simulink model "Steering"  (R2016a)
settings: Solver=FixedStepAuto  StartTime=0.0  StopTime=10  FixedStep=0.1  RelTol=1e-3
libraries: simulink x1
settings Model: Creator=krentzts  LastModifiedBy=krentzts
settings SolverCC: AlgebraicLoopSolver=LineSearch

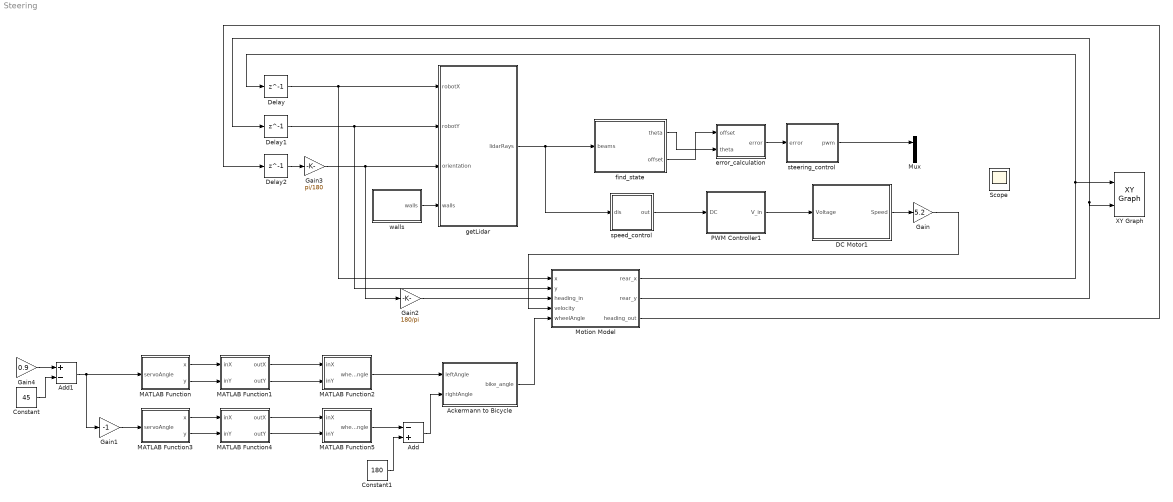
== system Steering ==
  Ackermann to Bicycle : MATLAB Function  TreatAsAtomicUnit=on
  Add : Sum  Inputs=-+
  Add1 : Sum  Inputs=+-
  Constant : Constant  Value=45
  Constant1 : Constant  Value=180
  DC Motor1 : Subsystem  mask{K=0.01, J=0.01, b=0.1, R=1, L=0.5}
      mask prompts: K "Ke (V/rad/sec), Kt (N.m/Amp)"; J "J (kg.m^2)"; b "b (N.m.s)"; R "R (Ohm)"; L "L (H)"
  Delay : Delay  DelayLength=1  InitialCondition=2
  Delay1 : Delay  DelayLength=1  InitialCondition=33
  Delay2 : Delay  DelayLength=1  InitialCondition=-20
  Gain : Gain  Gain=5.2
  Gain1 : Gain  Gain=-1
  Gain2 : Gain  Gain=180/pi
  Gain3 : Gain  Gain=pi/180
  Gain4 : Gain  Gain=0.9
  MATLAB Function : MATLAB Function  TreatAsAtomicUnit=on
  MATLAB Function1 : MATLAB Function  TreatAsAtomicUnit=on
  MATLAB Function2 : MATLAB Function  TreatAsAtomicUnit=on
  MATLAB Function3 : MATLAB Function  TreatAsAtomicUnit=on
  MATLAB Function4 : MATLAB Function  TreatAsAtomicUnit=on
  MATLAB Function5 : MATLAB Function  TreatAsAtomicUnit=on
  Motion Model : MATLAB Function  TreatAsAtomicUnit=on
  Mux : Mux  Inputs=2
  PWM Controller1 : Subsystem  mask{V=5}
      mask prompts: V "Maximum Voltage (V)"
  Scope : Scope
  XY Graph : simulink/Sinks/XY Graph  xmin=-1  xmax=1001  ymin=0  ymax=61  st=-1
  error_calculation : MATLAB Function  TreatAsAtomicUnit=on
  find_state : MATLAB Function  TreatAsAtomicUnit=on
  getLidar : MATLAB Function  TreatAsAtomicUnit=on
  speed_control : Stateflow chart  TreatAsAtomicUnit=on
  steering_control : Subsystem
  walls : MATLAB Function  TreatAsAtomicUnit=on
  wires:
  MATLAB Function/1(x) -> MATLAB Function1/1(inX)
  MATLAB Function/2(y) -> MATLAB Function1/2(inY)
  MATLAB Function1/1(outX) -> MATLAB Function2/1(inX)
  MATLAB Function1/2(outY) -> MATLAB Function2/2(inY)
  MATLAB Function2/1(wheelAngle) -> Ackermann to Bicycle/1(leftAngle)
  walls/1(walls) -> getLidar/4(walls)
  getLidar/1(lidarRays) -> find_state/1(beams), speed_control/1(dis)
  find_state/1(theta) -> error_calculation/2(theta)
  find_state/2(offset) -> error_calculation/1(offset)
  error_calculation/1(error) -> steering_control/1(error)
  PWM Controller1/1(V_in) -> DC Motor1/1(Voltage)
  DC Motor1/1(Speed) -> Gain/1
  Gain/1 -> Motion Model/4(velocity)
  Ackermann to Bicycle/1(bike_angle) -> Motion Model/5(wheelAngle)
  MATLAB Function3/1(x) -> MATLAB Function4/1(inX)
  MATLAB Function3/2(y) -> MATLAB Function4/2(inY)
  MATLAB Function4/1(outX) -> MATLAB Function5/1(inX)
  MATLAB Function4/2(outY) -> MATLAB Function5/2(inY)
  Gain1/1 -> MATLAB Function3/1(servoAngle)
  Add/1 -> Ackermann to Bicycle/2(rightAngle)
  MATLAB Function5/1(wheelAngle) -> Add/1
  Constant1/1 -> Add/2
  Gain2/1 -> Motion Model/3(heading_in)
  Motion Model/1(rear_x) -> Delay/1, XY Graph/1
  Motion Model/2(rear_y) -> XY Graph/2, Delay1/1
  Gain4/1 -> Add1/1
  Constant/1 -> Add1/2
  Add1/1 -> MATLAB Function/1(servoAngle), Gain1/1
  speed_control/1(out) -> PWM Controller1/1(DC)
  Delay2/1 -> Gain3/1
  Gain3/1 -> getLidar/3(orientation), Gain2/1
  Delay1/1 -> getLidar/2(robotY), Motion Model/2(y)
  Delay/1 -> getLidar/1(robotX), Motion Model/1(x)
  Motion Model/3(heading_out) -> Delay2/1
  steering_control/1(pwm) -> Mux/1

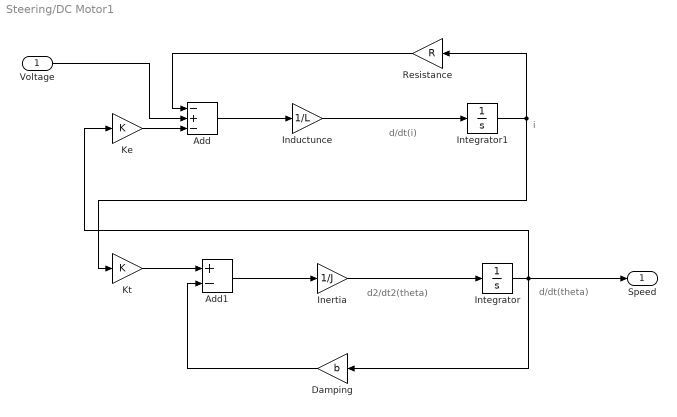
== system Steering/DC Motor1 ==
  note: d/dt(theta)
  note: i
  note: d2/dt2(theta)
  note: d/dt(i)
  Voltage : Inport
  Add : Sum  Inputs=-+-
  Add1 : Sum  Inputs=+-
  Damping : Gain  Gain=b
  Inductunce : Gain  Gain=1/L
  Inertia : Gain  Gain=1/J
  Integrator : Integrator
  Integrator1 : Integrator
  Ke : Gain  Gain=K
  Kt : Gain  Gain=K
  Resistance : Gain  Gain=R
  Speed : Outport
  wires:
  Kt/1 -> Add1/1
  Ke/1 -> Add/3
  Resistance/1 -> Add/1
  Voltage/1 -> Add/2
  Inductunce/1 -> Integrator1/1
  Integrator1/1 -> Resistance/1, Kt/1
  Inertia/1 -> Integrator/1
  Integrator/1 -> Speed/1, Damping/1, Ke/1
  Add/1 -> Inductunce/1
  Add1/1 -> Inertia/1
  Damping/1 -> Add1/2

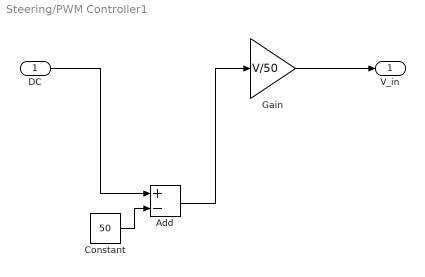
== system Steering/PWM Controller1 ==
  DC : Inport
  Add : Sum  Inputs=+-
  Constant : Constant  Value=50
  Gain : Gain  Gain=V/50
  V_in : Outport
  wires:
  Gain/1 -> V_in/1
  Constant/1 -> Add/2
  Add/1 -> Gain/1
  DC/1 -> Add/1

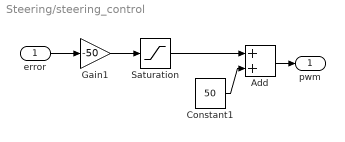
== system Steering/steering_control ==
  error : Inport
  Add : Sum
  Constant1 : Constant  Value=50
  Gain1 : Gain  Gain=-50
  Saturation : Saturate  UpperLimit=50  LowerLimit=-50
  pwm : Outport
  wires:
  error/1 -> Gain1/1
  Add/1 -> pwm/1
  Saturation/1 -> Add/1
  Gain1/1 -> Saturation/1
  Constant1/1 -> Add/2

== matlab function Steering/MATLAB Function1 ==
  data: inX input; outX output; inY input; outY output
function [outX,outY]  = pivotArm(inX,inY)
%#codegen
D = hypot(-1 - inX, -5 - inY);
theta1 = acosd((3.64^2 - 2^2 - D^2)/(-2*2*D));
theta2 = acosd((1+inX)/D);
thetaTotal = 360 - theta1 - theta2;

outLegAngle = thetaTotal - 180 + tand(1/2);

outX = -1 + sqrt(5)*cosd(outLegAngle);
outY = -5 + sqrt(5)*sind(outLegAngle);

== matlab function Steering/MATLAB Function ==
  data: x output; servoAngle input; y output
function [x,y] = servoHorn(servoAngle)
%#codegen

y = -7.07 + sind(270 - servoAngle);
x = 2.4813 + cosd(270 - servoAngle);

== matlab function Steering/MATLAB Function2 ==
  data: inX input; wheelAngle output; inY input
function wheelAngle = knuckle(inX,inY)
%#codegen
D = hypot(-10.5 - inX,0 - inY);
theta1 = acosd((9.2^2 - 1.5811^2 - D^2)/(-2*1.5811*D));
theta2 = acosd((10.5+inX)/D);
thetaTotal = 360 - theta1 - theta2;
wheelAngle = thetaTotal - 283.9 + 90;

== matlab function Steering/walls ==
  data: walls output
function walls = fcn()
walls=[1 1 1000 1;1 60 1000 60];
end

== matlab function Steering/getLidar ==
  data: robotX input; lidarRays output; robotY input; orientation input; walls input
function lidarRays = fcn(robotX,robotY,orientation,walls)

numLines = 512;
lidarRange = 60;

%Create rays matrix
lidarRays=zeros(numLines,2);
t = linspace(0,2*pi,numLines+1);
for i = 1:(length(t)-1);
    lidarRays(i,1) = lidarRange;
    lidarRays(i,2) = t(i);
end

[numWalls,~] = size(walls);
[numRays,~] = size(lidarRays);

%For each LIDAR ray...
for i = 1:numRays
    
    %Find its ending coordinate
    X = robotX + lidarRange*cos(t(i)+orientation);
    Y = robotY + lidarRange*sin(t(i)+orientation);
    
    %Find standard form of LIDAR ray
    R = [robotX robotY ; X Y];
    Q = inv(R)*[1;1];
    
    %For each wall...
    for j = 1:numWalls
        
        %Find standard form of wall
        P = [walls(j,1:2) ; walls(j,3:4)];
        O = inv(P)*[1;1];
        
        %Find intersection of wall and LIDAR ray
        INT = inv([Q';O'])*[1;1];
        intX = INT(1);  % x coordinate of intersection
        intY = INT(2);  % y coordinate of intersection
        
        %Check that intersection actually occurs within the
        %bounds of the LIDAR ray and wall
        if ((isBetween(intY,robotY,Y) == 1) && ...
            (isBetween(intX,robotX,X) == 1) && ...
            (isBetween(intX,walls(j,1),walls(j,3)) == 1) && ...
            (isBetween(intY,walls(j,2),walls(j,4)) == 1))
%             disp('INTERSECTION')
            temp = hypot((intX-robotX),(intY-robotY));
            
            %Clip ranges beyond max sensitivity
            if(temp > lidarRange)
                temp = lidarRange;
            end
            
            %Only store the minimum range for each wall
            if (lidarRays(i,1) > temp)
                lidarRays(i,1) = temp;
            end
        else
%             disp('NOPE')
        end
    end
end

== matlab function Steering/find_state ==
  data: theta output; beams input; offset output
function [theta,offset]  = fcn(beams)
step=2*pi/length(beams);
theta=0;
[~,minimum]=min(beams(:,1));
[~,min_left]=min(beams(2:(length(beams)/2),1));
[~,min_right]=min(beams((length(beams)/2)+2:end,1));
firstBeam = beams(1,1);
rearBeam = beams(129,1)

%if minimum is in front or behind then

disp((size(beams)));
if (firstBeam < rearBeam)
    if minimum<=length(beams)/2
        theta=(pi/2)-(minimum-1)*step;
    else
        theta=-((pi/2)-(length(beams)+1-minimum)*step);
    end
elseif (firstBeam > rearBeam)
    if minimum<=length(beams)/2
        theta=-((pi/2)-((length(beams)/2+1)-minimum)*step);
    else
        theta=(pi/2)-(minimum-(length(beams)/2+1.5))*step;
    end
end

if minimum<=length(beams)/2
    x=beams(minimum+(length(beams)/2),1);
    y=beams(minimum,1);
else
    x=beams(minimum,1);
    y=beams(minimum-(length(beams)/2),1);
end
offset=(x+y)/2-y;
end

== matlab function Steering/error_calculation ==
  data: offset input; error output; theta input
function error = fcn(offset,theta)
L=3;
error=offset+L*sin(theta);
%positive error means turn right

== stateflow chart Steering/speed_control ==
  state forward
    du: PWM=80;
  state stop
    du: PWM=50;
  state back_right
    du: PWM = 40
  state back_left
    du: PWM = 40
  state straighten_left
    du: PWM = 60
  state straighten_right
    du: PWM = 60
  (default) -> forward
  forward -> stop : [dis(1,1)<0.25]
  data: dis input; out output

== matlab function Steering/Motion Model ==
  data: x input; rear_x output; y input; heading_in input; velocity input; wheelAngle input; rear_y output; heading_out output
function [rear_x,rear_y,heading_out] = fcn(x,y,heading_in,velocity,wheelAngle)
%#codegen
%heading_in=rad2deg(heading_in);
timestep = 0.1; %seconds
wheelBase = 16;
rw.x = x;
rw.y = y;
fw.x = rw.x+cosd(heading_in)*wheelBase;
fw.y = rw.y+sind(heading_in)*wheelBase;

if(wheelAngle == 90)
    wheelAngle = wheelAngle + 0.0001;
end
alpha = wheelAngle;
turningRadius = tand(alpha)*wheelBase;
arcLength = velocity * timestep;
theta = arcLength / turningRadius;
theta = theta * (180/pi);

dx = turningRadius - (cosd(theta)*turningRadius);
dy = sind(theta)*turningRadius;

rw.x = rw.x + cosd(heading_in)*dx + cosd(heading_in)*dy;
rw.y = rw.y + sind(heading_in)*dx + sind(heading_in)*dy;
heading_out = heading_in - theta;
rear_x=rw.x;
rear_y=rw.y;

== matlab function Steering/Ackermann to Bicycle ==
  data: leftAngle input; bike_angle output; rightAngle input
function bike_angle  = fcn(leftAngle,rightAngle)
%#codegen
    wheelbase = 32;
    wheelwidth = 25;
    if (leftAngle < 89.3)   
        fraction = (2*wheelwidth*tand(rightAngle))/(tand(leftAngle)-tand(rightAngle));
        fraction = (fraction + wheelwidth)/wheelbase;
        bike_angle = atand(fraction);
    elseif (leftAngle > 90.7)
        temp = rightAngle;
        rightAngle = leftAngle-180;
        leftAngle = temp-180;
        fraction = (2*wheelwidth*tand(rightAngle))/(tand(leftAngle)-tand(rightAngle));
        fraction = (fraction + wheelwidth)/wheelbase;
        bike_angle = 180 - atand(fraction);
    else
        bike_angle = 90;
    end
end

== matlab function Steering/MATLAB Function3 ==
  data: x output; servoAngle input; y output
function [x,y] = servoHorn(servoAngle)
%#codegen

y = -7.07 + sind(270 - servoAngle);
x = 2.4813 + cosd(270 - servoAngle);

== matlab function Steering/MATLAB Function4 ==
  data: inX input; outX output; inY input; outY output
function [outX,outY]  = pivotArm(inX,inY)
%#codegen
D = hypot(-1 - inX, -5 - inY);
theta1 = acosd((3.64^2 - 2^2 - D^2)/(-2*2*D));
theta2 = acosd((1+inX)/D);
thetaTotal = 360 - theta1 - theta2;

outLegAngle = thetaTotal - 180 + tand(1/2);

outX = -1 + sqrt(5)*cosd(outLegAngle);
outY = -5 + sqrt(5)*sind(outLegAngle);

== matlab function Steering/MATLAB Function5 ==
  data: inX input; wheelAngle output; inY input
function wheelAngle = knuckle(inX,inY)
%#codegen
D = hypot(-10.5 - inX,0 - inY);
theta1 = acosd((9.2^2 - 1.5811^2 - D^2)/(-2*1.5811*D));
theta2 = acosd((10.5+inX)/D);
thetaTotal = 360 - theta1 - theta2;
wheelAngle = thetaTotal - 283.9 + 90;
